simulink model "Test2uCRG"  (R2022b)
settings: Solver=VariableStepAuto  StartTime=0.0  StopTime=60  FixedStep=0.01  RelTol=1e-3
undefined symbols (not defined in the file): LF
libraries: instrumentseriallib x2, instrumentlib x2
settings Model: Creator=Jovani  LastModifiedBy=Jovani
settings OptimizationCC: DefaultParameterBehavior=Inlined  EnhancedBackFolding=on  PassReuseOutputArgsAs=Individual arguments  ZeroExternalMemoryAtStartup=off  ZeroInternalMemoryAtStartup=off  MaxStackSize=64  OptimizeBlockOrder=speed  DifferentSizesBufferReuse=on  OptimizationCustomize=off  EfficientTunableParamExpr=on
settings DebuggingCC: ParameterTunabilityLossMsg=error
settings HardwareCC: ProdBitPerLong=64  ProdLargestAtomicFloat=None  ProdHWDeviceType=AMD->Athlon 64  UseEmbeddedCoderFeatures=off  UseSimulinkCoderFeatures=off
settings SFSimCC: MATLABDynamicMemAlloc=off
settings RTWCC: Description=Embedded Coder  SystemTargetFile=ert.tlc  TemplateMakefile=ert_default_tmf  Toolchain=Arduino AVR  BuildConfiguration=Faster Runs
settings CodeAppCC: ForceParamTrailComments=on  IgnoreCustomStorageClasses=off  OperatorAnnotations=on  SimulinkDataObjDesc=on  SFDataObjDesc=on  InsertBlockDesc=on
settings ERTTargetCC: SupportContinuousTime=on  SupportNonInlinedSFcns=on  ExtModeTransport=3  ExtModeStaticAlloc=on  ExtModeStaticAllocSize=250  ExtModeMexFile=ext_xcp  ExtModeIntrfLevel=Level2 - Open  InlinedParameterPlacement=NonHierarchical  ERTCustomFileTemplate=example_file_process.tlc

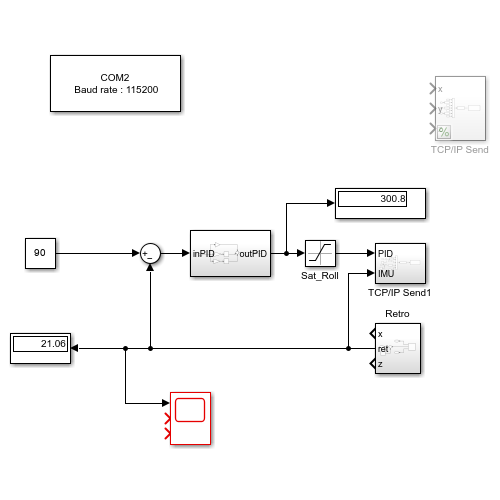
[thumbnail: Simulink's stored preview of the top-level diagram]
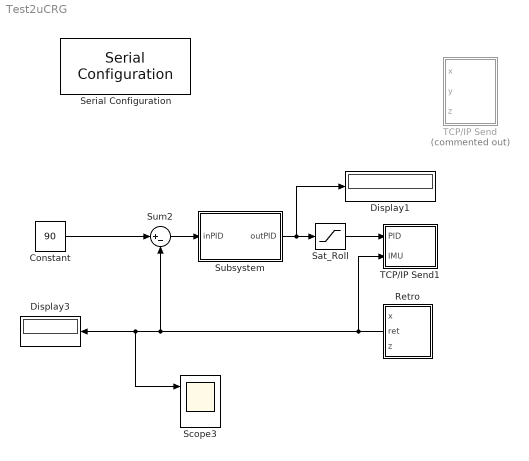
== system Test2uCRG ==
  Constant : Constant  Value=90
  Display1 : Display
  Display3 : Display
  Retro : Subsystem
  Sat_Roll : Saturate  UpperLimit=1000  LowerLimit=-1000
  Scope3 : Scope  NumInputPorts=3
  Serial Configuration : instrumentseriallib/Serial Configuration  Priority=-200000  PortSel=COM2  Port=COM2  ComPort=COM2  BaudRate=115200  DataBits=8  Parity=none  StopBits=1  ByteOrder=little-endian  FlowControl=none  Timeout=10  SimulateUsing=Interpreted execution  BlockInModel=on  aMode=1
  Subsystem : Subsystem
  Sum2 : Sum  Inputs=|+-
  TCP/IP Send : Subsystem  Commented=on
  TCP/IP Send1 : Subsystem
  wires:
  Constant/1 -> Sum2/1
  Sum2/1 -> Subsystem/1(inPID)
  Subsystem/1(outPID) -> Display1/1, Sat_Roll/1
  Retro/2(ret) -> TCP/IP Send1/2(IMU), Sum2/2, Scope3/1, Display3/1
  Sat_Roll/1 -> TCP/IP Send1/1(PID)

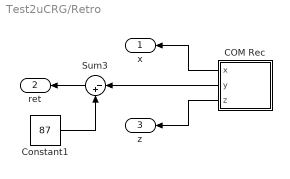
== system Test2uCRG/Retro ==
  COM Rec : Subsystem
  Constant1 : Constant  Value=87
  Sum3 : Sum  Inputs=|-+
  x : Outport
  ret : Outport  Port=2
  z : Outport  Port=3
  wires:
  Sum3/1 -> ret/1
  Constant1/1 -> Sum3/2
  COM Rec/3(z) -> z/1
  COM Rec/2(y) -> Sum3/1
  COM Rec/1(x) -> x/1

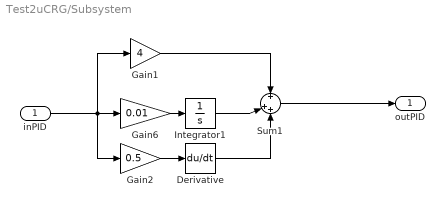
== system Test2uCRG/Subsystem ==
  inPID : Inport
  Derivative : Derivative
  Gain1 : Gain  Gain=4
  Gain2 : Gain  Gain=0.5
  Gain6 : Gain  Gain=0.01
  Integrator1 : Integrator
  Sum1 : Sum  Inputs=+|++
  outPID : Outport
  wires:
  Derivative/1 -> Sum1/3
  Integrator1/1 -> Sum1/2
  inPID/1 -> Gain1/1, Gain2/1, Gain6/1
  Gain2/1 -> Derivative/1
  Sum1/1 -> outPID/1
  Gain6/1 -> Integrator1/1
  Gain1/1 -> Sum1/1

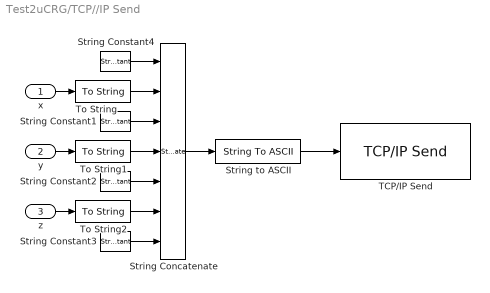
== system Test2uCRG/TCP//IP Send ==
  x : Inport
  y : Inport  Port=2
  z : Inport  Port=3
  String Concatenate : StringConcatenate  Inputs=7
  String Constant1 : StringConstant  String="\"y\""
  String Constant2 : StringConstant  String="\"z\""
  String Constant3 : StringConstant  String="\"r\""
  String Constant4 : StringConstant  String="\"x\""
  String to ASCII : StringToASCII
  TCP/IP Send : instrumentlib/TCP//IP Send  Host=192.168.100.31  Port=22333  ByteOrder=little-endian  EnableBlockingMode=on  Timeout=10  TransferDelay=on  SimulateUsing=Interpreted execution
  To String : ToString
  To String1 : ToString
  To String2 : ToString
  wires:
  String Concatenate/1 -> String to ASCII/1
  To String/1 -> String Concatenate/2
  String to ASCII/1 -> TCP/IP Send/1
  To String2/1 -> String Concatenate/6
  To String1/1 -> String Concatenate/4
  String Constant2/1 -> String Concatenate/5
  String Constant1/1 -> String Concatenate/3
  String Constant3/1 -> String Concatenate/7
  String Constant4/1 -> String Concatenate/1
  z/1 -> To String2/1
  x/1 -> To String/1
  y/1 -> To String1/1

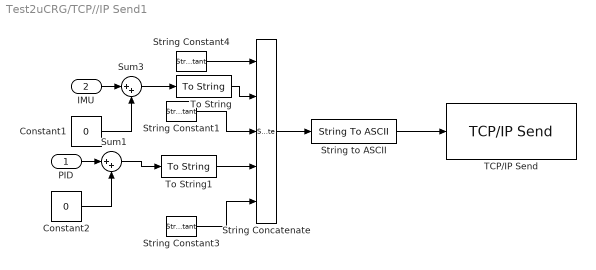
== system Test2uCRG/TCP//IP Send1 ==
  PID : Inport
  IMU : Inport  Port=2
  Constant1 : Constant  Value=0
  Constant2 : Constant  Value=0
  String Concatenate : StringConcatenate  Inputs=5
  String Constant1 : StringConstant  String="\"y\""
  String Constant3 : StringConstant  String="\"r\""
  String Constant4 : StringConstant  String="\"x\""
  String to ASCII : StringToASCII
  Sum1 : Sum  Inputs=|++
  Sum3 : Sum  Inputs=|++
  TCP/IP Send : instrumentlib/TCP//IP Send  Host=192.168.100.31  Port=22333  ByteOrder=little-endian  EnableBlockingMode=on  Timeout=10  TransferDelay=on  SimulateUsing=Interpreted execution
  To String : ToString
  To String1 : ToString
  wires:
  String Concatenate/1 -> String to ASCII/1
  To String/1 -> String Concatenate/2
  String to ASCII/1 -> TCP/IP Send/1
  String Constant4/1 -> String Concatenate/1
  IMU/1 -> Sum3/1
  Constant1/1 -> Sum3/2
  Sum3/1 -> To String/1
  String Constant1/1 -> String Concatenate/3
  Constant2/1 -> Sum1/2
  Sum1/1 -> To String1/1
  PID/1 -> Sum1/1
  To String1/1 -> String Concatenate/4
  String Constant3/1 -> String Concatenate/5

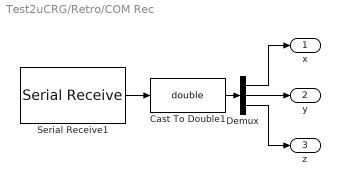
== system Test2uCRG/Retro/COM Rec ==
  Cast To Double1 : DataTypeConversion  OutDataTypeStr=double  SaturateOnIntegerOverflow=off  RndMeth=Floor
  Demux : Demux  Outputs=3
  Serial Receive1 : instrumentseriallib/Serial Receive  PortSel=COM2  Port=COM2  ComPort=COM2  DataType=single  SaveDataType=uint8  ToggleHeader=on  Header='z'  ToggleTerminator=on  Terminator=LF ('\n')  CustomTerminator=[]  InputFormat=Column major  ToggleDataSize=on  DataSize="[1  3]"  EnableBlockingMode=on  ActionDataUnavailable=Output last received value  ActionWhenDataUnavailable=Output last received value  CustomValue=0  SampleTime=0.05  SimulateUsing=Interpreted execution  BlockInModel=on  aMode=1
  x : Outport
  y : Outport  Port=2
  z : Outport  Port=3
  wires:
  Serial Receive1/1 -> Cast To Double1/1
  Cast To Double1/1 -> Demux/1
  Demux/1 -> x/1
  Demux/2 -> y/1
  Demux/3 -> z/1
